simulink model "Lab7_Kho_Nguyen_Soh_AbdulKadir_simulink"  (R2021a)
settings: Solver=VariableStepAuto  StartTime=0.0  StopTime=10  MinStep=0.01  RelTol=1e-3
libraries: pid_lib x10, cstblocks x5
settings Model: Creator=fayeed  LastModifiedBy=kkqi_
settings SolverCC: AlgebraicLoopSolver=TrustRegion
settings DebuggingCC: SFMachineParentedDataDiag=warning

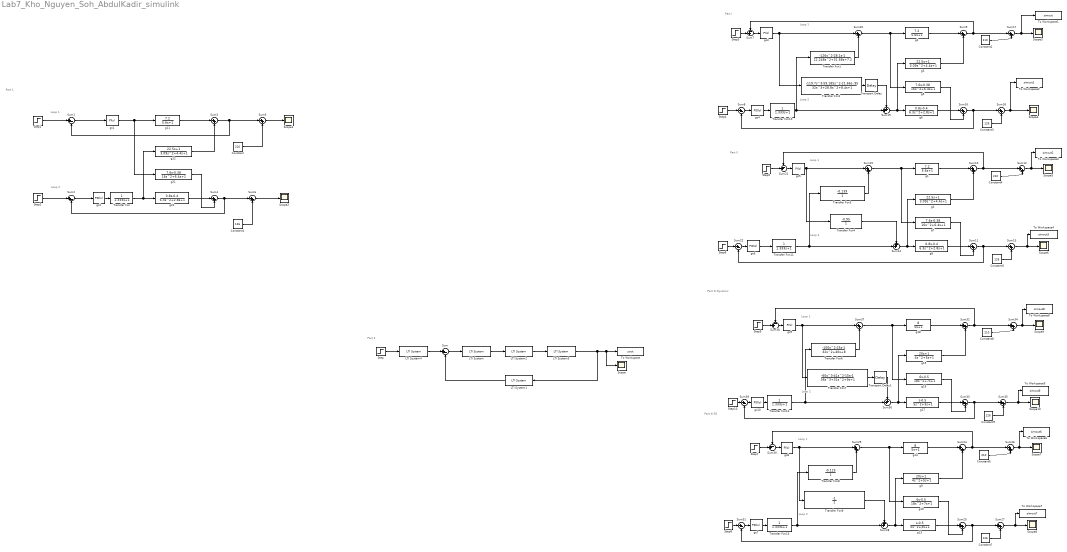
== system Lab7_Kho_Nguyen_Soh_AbdulKadir_simulink ==
  note: Part 1
  note: Part 3
  note: Loop 1
  note: Loop 2
  note: Part II
  note: Loop 2
  note: Loop 2
  note: Loop 1
  note: Loop 2
  note: Part I
  note: Loop 2
  note: Loop 1
  note: Loop 1
  note: Part III SS
  note: Part III Dynamic
  note: Loop 1
  Constant{,2,4,6,8} (5 alike) : Constant  Value=210
  Constant{1,3,5,7,9} (5 alike) : Constant  Value=126
  LTI System : cstblocks/LTI System  sys=Gc  IC=[]
  LTI System1 : cstblocks/LTI System  sys=WT  IC=[]
  LTI System2 : cstblocks/LTI System  sys=V  IC=[]
  LTI System3 : cstblocks/LTI System  sys=G  IC=[]
  LTI System4 : cstblocks/LTI System  sys=WT  IC=[]
  Scope{,1..10} (11 alike) : Scope
  Step : Step  Time=0  Before=[0,0,0]  After=[0,0,-10]  SampleTime=0
  Step{1,3,5,7,9} (5 alike) : Step  Time=0  After=15  SampleTime=0
  Step{2,4,6,8,10} (5 alike) : Step  Time=0  After=0  SampleTime=0
  Sum{,1..2,8,22,31,39} (7 alike) : Sum  Inputs=|+-
  Sum{3..6,9..13,15..18,20,24..27,29,32..35,37} (24 alike) : Sum  Inputs=|++
  Sum{14,19,28,36} (4 alike) : Sum  Inputs=++|
  Sum{7,21,30,38} (4 alike) : Sum  Inputs=-+|
  To Workspace : ToWorkspace  VariableName=yout  SampleTime=-1
  To Workspace1 : ToWorkspace  VariableName=simout  SampleTime=-1
  To Workspace2 : ToWorkspace  VariableName=simout1  SampleTime=-1
  To Workspace3 : ToWorkspace  VariableName=simout2  SampleTime=-1
  To Workspace4 : ToWorkspace  VariableName=simout3  SampleTime=-1
  To Workspace6 : ToWorkspace  VariableName=simout6  SampleTime=-1
  To Workspace7 : ToWorkspace  VariableName=simout7  SampleTime=-1
  To Workspace8 : ToWorkspace  VariableName=simout8  SampleTime=-1
  To Workspace9 : ToWorkspace  VariableName=simout9  SampleTime=-1
  Transfer Fcn{,10..13} (5 alike) : TransferFcn  Denominator=[1.333 1]
  Transfer Fcn1 : TransferFcn  Numerator=[-126 -28.1 -1]  Denominator=[22.248 31.68 7.2]
  Transfer Fcn2 : TransferFcn  Numerator=[-119.7 -59.185 -21.66 -.95]  Denominator=[32 28.8 8.4 1]
  Transfer Fcn3 : TransferFcn  Numerator=[-0.139]  Denominator=[1]
  Transfer Fcn4 : TransferFcn  Numerator=[-0.95]  Denominator=[1]
  Transfer Fcn6 : TransferFcn  Numerator=[-100 -25 -1]  Denominator=[32 40 8]
  Transfer Fcn7 : TransferFcn  Numerator=[-60 -41 -15 -1]  Denominator=[36 31 9 1]
  Transfer Fcn8 : TransferFcn  Numerator=[-0.125]  Denominator=[1]
  Transfer Fcn9 : TransferFcn  Numerator=[-1]  Denominator=[1]
  Transport Delay : TransportDelay  DelayTime=36
  Transport Delay1 : TransportDelay  DelayTime=20
  g1 : TransferFcn  Numerator=[7.2]  Denominator=[5.6 1]
  g10 : TransferFcn  Numerator=[6 -0.5]  Denominator=[18 7 1]
  g11 : TransferFcn  Numerator=[7.2]  Denominator=[5.6 1]
  g12 : TransferFcn  Numerator=[22.5 1]  Denominator=[3.09 4.4 1]
  g13 : TransferFcn  Numerator=[1 -0.5]  Denominator=[5 3 1 ]
  g14 : TransferFcn  Numerator=[8]  Denominator=[5 1]
  g15 : TransferFcn  Numerator=[20 1]  Denominator=[4 5 1]
  g16 : TransferFcn  Numerator=[6 -0.5]  Denominator=[18 7 1]
  g17 : TransferFcn  Numerator=[1 -0.5]  Denominator=[5 3 1 ]
  g18 : TransferFcn  Numerator=[8]  Denominator=[5 1]
  g2 : TransferFcn  Numerator=[7.2]  Denominator=[5.6 1]
  g21 : TransferFcn  Numerator=[7.6 -0.38]  Denominator=[16 6.4 1]
  g22 : TransferFcn  Numerator=[0.8 -0.4]  Denominator=[6.3 2.8 1]
  g3 : TransferFcn  Numerator=[22.5 1]  Denominator=[3.09 4.4 1]
  g4 : TransferFcn  Numerator=[22.5 1]  Denominator=[3.09 4.4 1]
  g5 : TransferFcn  Numerator=[7.6 -0.38]  Denominator=[16 6.4 1]
  g6 : TransferFcn  Numerator=[0.8 -0.4]  Denominator=[6.3 2.8 1]
  g7 : TransferFcn  Numerator=[7.6 -0.38]  Denominator=[16 6.4 1]
  g8 : TransferFcn  Numerator=[0.8 -0.4]  Denominator=[6.3 2.8 1]
  g9 : TransferFcn  Numerator=[20 1]  Denominator=[4 5 1]
  gc1 : pid_lib/PID Controller  Controller=PI  Form=Ideal  TimeDomain=Continuous-time  UseExternalTs=off  SampleTime=-1  IntegratorMethod=Forward Euler  FilterMethod=Forward Euler  ControllerParametersSource=internal  P=0.778  I=0.1779  D=0  UseFilter=on  N=100  TunerSelectOption=Transfer Function Based (PID Tuner App)  InitialConditionSource=internal  InitialConditionForIntegrator=0  InitialConditionForFilter=0  DifferentiatorICPrevScaledInput=0  ExternalReset=none  TrackingMode=off  Kt=1  LimitOutput=off  SatLimitsSource=internal  UpperSaturationLimit=inf  LowerSaturationLimit=-inf  LinearizeAsGain=on  AntiWindupMode=none  Kb=1  POutMin=[]  POutMax=[]  IOutMin=[]  IOutMax=[]  DOutMin=[]  DOutMax=[]  NOutMin=[]  NOutMax=[]  SumOutMin=[]  SumOutMax=[]  SaturationOutMin=[]  SaturationOutMax=[]  PParamMin=[]  PParamMax=[]  IParamMin=[]  IParamMax=[]  DParamMin=[]  DParamMax=[]  NParamMin=[]  NParamMax=[]  KbParamMin=[]  KbParamMax=[]  KtParamMin=[]  KtParamMax=[]  KbOutMin=[]  KbOutMax=[]  KtOutMin=[]  KtOutMax=[]  IntegratorOutMin=[]  IntegratorOutMax=[]  FilterOutMin=[]  FilterOutMax=[]  SumI1OutMin=[]  SumI1OutMax=[]  SumI2OutMin=[]  SumI2OutMax=[]  SumI3OutMin=[]  SumI3OutMax=[]  SumI4OutMin=[]  SumI4OutMax=[]  SumDOutMin=[]  SumDOutMax=[]  DifferentiatorOutMin=[]  DifferentiatorOutMax=[]  FilterDiffOutCoefMin=[]  FilterDiffOutCoefMax=[]  ReciprocalOutMin=[]  ReciprocalOutMax=[]  SumDenOutMin=[]  SumDenOutMax=[]  SumNumOutMin=[]  SumNumOutMax=[]  DivideOutMin=[]  DivideOutMax=[]  UdiffTsProdOutMin=[]  UdiffTsProdOutMax=[]  NTsProdOutMin=[]  NTsProdOutMax=[]  UintegralTsProdOutMin=[]  UintegralTsProdOutMax=[]  UngainTsProdOutMin=[]  UngainTsProdOutMax=[]  IntegratorContinuousStateAttributes=''  IntegratorStateMustResolveToSignalObject=off  IntegratorRTWStateStorageClass=Auto  FilterContinuousStateAttributes=''  FilterStateMustResolveToSignalObject=off  FilterRTWStateStorageClass=Auto  ParallelPVariant=Passthrough  IdealPVariant=InternalParameters  IVariant=InternalParameters  DVariant=Disabled  IntegratorVariant=Continuous  SatVariant=Disabled  AWVariant=Passthrough  PCopyVariant=Disabled  TRVariant=Disabled  FdbkBlocksVariant=Forward  IdealPFdbkVariant=Disabled  SatFdbkVariant=Disabled  DerivativeFilterVariant=Disabled  NVariant=Disabled  NCopyVariant=Disabled_SignalSpec  FilterICVariant=Disabled  IntegratorICVariant=InternalICs  ExternalResetVariant=Disabled  TRSumVariant=Passthrough  SumFdbkVariant=Disabled  SumVariant=Sum_PI  TsampFilterVariant=InternalTs  TsampNgainVariant=Passthrough  TsampIntegralVariant=Passthrough  ExternalSaturationOutDataTypeStr=Inherit: Same as second input
  gc{2,4,6..7,10} (5 alike) : pid_lib/PID Controller  Controller=PID  Form=Ideal  TimeDomain=Continuous-time  UseExternalTs=off  SampleTime=-1  IntegratorMethod=Forward Euler  FilterMethod=Forward Euler  ControllerParametersSource=internal  P=-0.778  I=0.357  D=2.25  UseFilter=on  N=100  TunerSelectOption=Transfer Function Based (PID Tuner App)  InitialConditionSource=internal  InitialConditionForIntegrator=0  InitialConditionForFilter=0  DifferentiatorICPrevScaledInput=0  ExternalReset=none  TrackingMode=off  Kt=1  LimitOutput=off  SatLimitsSource=internal  UpperSaturationLimit=inf  LowerSaturationLimit=-inf  LinearizeAsGain=on  AntiWindupMode=none  Kb=1  POutMin=[]  POutMax=[]  IOutMin=[]  IOutMax=[]  DOutMin=[]  DOutMax=[]  NOutMin=[]  NOutMax=[]  SumOutMin=[]  SumOutMax=[]  SaturationOutMin=[]  SaturationOutMax=[]  PParamMin=[]  PParamMax=[]  IParamMin=[]  IParamMax=[]  DParamMin=[]  DParamMax=[]  NParamMin=[]  NParamMax=[]  KbParamMin=[]  KbParamMax=[]  KtParamMin=[]  KtParamMax=[]  KbOutMin=[]  KbOutMax=[]  KtOutMin=[]  KtOutMax=[]  IntegratorOutMin=[]  IntegratorOutMax=[]  FilterOutMin=[]  FilterOutMax=[]  SumI1OutMin=[]  SumI1OutMax=[]  SumI2OutMin=[]  SumI2OutMax=[]  SumI3OutMin=[]  SumI3OutMax=[]  SumI4OutMin=[]  SumI4OutMax=[]  SumDOutMin=[]  SumDOutMax=[]  DifferentiatorOutMin=[]  DifferentiatorOutMax=[]  FilterDiffOutCoefMin=[]  FilterDiffOutCoefMax=[]  ReciprocalOutMin=[]  ReciprocalOutMax=[]  SumDenOutMin=[]  SumDenOutMax=[]  SumNumOutMin=[]  SumNumOutMax=[]  DivideOutMin=[]  DivideOutMax=[]  UdiffTsProdOutMin=[]  UdiffTsProdOutMax=[]  NTsProdOutMin=[]  NTsProdOutMax=[]  UintegralTsProdOutMin=[]  UintegralTsProdOutMax=[]  UngainTsProdOutMin=[]  UngainTsProdOutMax=[]  IntegratorContinuousStateAttributes=''  IntegratorStateMustResolveToSignalObject=off  IntegratorRTWStateStorageClass=Auto  FilterContinuousStateAttributes=''  FilterStateMustResolveToSignalObject=off  FilterRTWStateStorageClass=Auto  ParallelPVariant=Passthrough  IdealPVariant=InternalParameters  IVariant=InternalParameters  DVariant=InternalParameters  IntegratorVariant=Continuous  SatVariant=Disabled  AWVariant=Passthrough  PCopyVariant=Disabled  TRVariant=Disabled  FdbkBlocksVariant=Forward  IdealPFdbkVariant=Disabled  SatFdbkVariant=Disabled  DerivativeFilterVariant=ContFilter  NVariant=InternalParameters  NCopyVariant=Disabled  FilterICVariant=InternalICsFilter  IntegratorICVariant=InternalICs  ExternalResetVariant=Disabled  TRSumVariant=Passthrough  SumFdbkVariant=Disabled  SumVariant=Sum_PID  TsampFilterVariant=InternalTs  TsampNgainVariant=Passthrough  TsampIntegralVariant=Passthrough  ExternalSaturationOutDataTypeStr=Inherit: Same as second input
  gc3 : pid_lib/PID Controller  Controller=PI  Form=Ideal  TimeDomain=Continuous-time  UseExternalTs=off  SampleTime=-1  IntegratorMethod=Forward Euler  FilterMethod=Forward Euler  ControllerParametersSource=internal  P=0.778  I=0.1779  D=0  UseFilter=on  N=100  TunerSelectOption=Transfer Function Based (PID Tuner App)  InitialConditionSource=internal  InitialConditionForIntegrator=0  InitialConditionForFilter=0  DifferentiatorICPrevScaledInput=0  ExternalReset=none  TrackingMode=off  Kt=1  LimitOutput=off  SatLimitsSource=internal  UpperSaturationLimit=inf  LowerSaturationLimit=-inf  LinearizeAsGain=on  AntiWindupMode=none  Kb=1  POutMin=[]  POutMax=[]  IOutMin=[]  IOutMax=[]  DOutMin=[]  DOutMax=[]  NOutMin=[]  NOutMax=[]  SumOutMin=[]  SumOutMax=[]  SaturationOutMin=[]  SaturationOutMax=[]  PParamMin=[]  PParamMax=[]  IParamMin=[]  IParamMax=[]  DParamMin=[]  DParamMax=[]  NParamMin=[]  NParamMax=[]  KbParamMin=[]  KbParamMax=[]  KtParamMin=[]  KtParamMax=[]  KbOutMin=[]  KbOutMax=[]  KtOutMin=[]  KtOutMax=[]  IntegratorOutMin=[]  IntegratorOutMax=[]  FilterOutMin=[]  FilterOutMax=[]  SumI1OutMin=[]  SumI1OutMax=[]  SumI2OutMin=[]  SumI2OutMax=[]  SumI3OutMin=[]  SumI3OutMax=[]  SumI4OutMin=[]  SumI4OutMax=[]  SumDOutMin=[]  SumDOutMax=[]  DifferentiatorOutMin=[]  DifferentiatorOutMax=[]  FilterDiffOutCoefMin=[]  FilterDiffOutCoefMax=[]  ReciprocalOutMin=[]  ReciprocalOutMax=[]  SumDenOutMin=[]  SumDenOutMax=[]  SumNumOutMin=[]  SumNumOutMax=[]  DivideOutMin=[]  DivideOutMax=[]  UdiffTsProdOutMin=[]  UdiffTsProdOutMax=[]  NTsProdOutMin=[]  NTsProdOutMax=[]  UintegralTsProdOutMin=[]  UintegralTsProdOutMax=[]  UngainTsProdOutMin=[]  UngainTsProdOutMax=[]  IntegratorContinuousStateAttributes=''  IntegratorStateMustResolveToSignalObject=off  IntegratorRTWStateStorageClass=Auto  FilterContinuousStateAttributes=''  FilterStateMustResolveToSignalObject=off  FilterRTWStateStorageClass=Auto  ParallelPVariant=Passthrough  IdealPVariant=InternalParameters  IVariant=InternalParameters  DVariant=Disabled  IntegratorVariant=Continuous  SatVariant=Disabled  AWVariant=Passthrough  PCopyVariant=Disabled  TRVariant=Disabled  FdbkBlocksVariant=Forward  IdealPFdbkVariant=Disabled  SatFdbkVariant=Disabled  DerivativeFilterVariant=Disabled  NVariant=Disabled  NCopyVariant=Disabled_SignalSpec  FilterICVariant=Disabled  IntegratorICVariant=InternalICs  ExternalResetVariant=Disabled  TRSumVariant=Passthrough  SumFdbkVariant=Disabled  SumVariant=Sum_PI  TsampFilterVariant=InternalTs  TsampNgainVariant=Passthrough  TsampIntegralVariant=Passthrough  ExternalSaturationOutDataTypeStr=Inherit: Same as second input
  gc5 : pid_lib/PID Controller  Controller=PI  Form=Ideal  TimeDomain=Continuous-time  UseExternalTs=off  SampleTime=-1  IntegratorMethod=Forward Euler  FilterMethod=Forward Euler  ControllerParametersSource=internal  P=.0778  I=.1779  D=0  UseFilter=on  N=100  TunerSelectOption=Transfer Function Based (PID Tuner App)  InitialConditionSource=internal  InitialConditionForIntegrator=0  InitialConditionForFilter=0  DifferentiatorICPrevScaledInput=0  ExternalReset=none  TrackingMode=off  Kt=1  LimitOutput=off  SatLimitsSource=internal  UpperSaturationLimit=inf  LowerSaturationLimit=-inf  LinearizeAsGain=on  AntiWindupMode=none  Kb=1  POutMin=[]  POutMax=[]  IOutMin=[]  IOutMax=[]  DOutMin=[]  DOutMax=[]  NOutMin=[]  NOutMax=[]  SumOutMin=[]  SumOutMax=[]  SaturationOutMin=[]  SaturationOutMax=[]  PParamMin=[]  PParamMax=[]  IParamMin=[]  IParamMax=[]  DParamMin=[]  DParamMax=[]  NParamMin=[]  NParamMax=[]  KbParamMin=[]  KbParamMax=[]  KtParamMin=[]  KtParamMax=[]  KbOutMin=[]  KbOutMax=[]  KtOutMin=[]  KtOutMax=[]  IntegratorOutMin=[]  IntegratorOutMax=[]  FilterOutMin=[]  FilterOutMax=[]  SumI1OutMin=[]  SumI1OutMax=[]  SumI2OutMin=[]  SumI2OutMax=[]  SumI3OutMin=[]  SumI3OutMax=[]  SumI4OutMin=[]  SumI4OutMax=[]  SumDOutMin=[]  SumDOutMax=[]  DifferentiatorOutMin=[]  DifferentiatorOutMax=[]  FilterDiffOutCoefMin=[]  FilterDiffOutCoefMax=[]  ReciprocalOutMin=[]  ReciprocalOutMax=[]  SumDenOutMin=[]  SumDenOutMax=[]  SumNumOutMin=[]  SumNumOutMax=[]  DivideOutMin=[]  DivideOutMax=[]  UdiffTsProdOutMin=[]  UdiffTsProdOutMax=[]  NTsProdOutMin=[]  NTsProdOutMax=[]  UintegralTsProdOutMin=[]  UintegralTsProdOutMax=[]  UngainTsProdOutMin=[]  UngainTsProdOutMax=[]  IntegratorContinuousStateAttributes=''  IntegratorStateMustResolveToSignalObject=off  IntegratorRTWStateStorageClass=Auto  FilterContinuousStateAttributes=''  FilterStateMustResolveToSignalObject=off  FilterRTWStateStorageClass=Auto  ParallelPVariant=Passthrough  IdealPVariant=InternalParameters  IVariant=InternalParameters  DVariant=Disabled  IntegratorVariant=Continuous  SatVariant=Disabled  AWVariant=Passthrough  PCopyVariant=Disabled  TRVariant=Disabled  FdbkBlocksVariant=Forward  IdealPFdbkVariant=Disabled  SatFdbkVariant=Disabled  DerivativeFilterVariant=Disabled  NVariant=Disabled  NCopyVariant=Disabled_SignalSpec  FilterICVariant=Disabled  IntegratorICVariant=InternalICs  ExternalResetVariant=Disabled  TRSumVariant=Passthrough  SumFdbkVariant=Disabled  SumVariant=Sum_PI  TsampFilterVariant=InternalTs  TsampNgainVariant=Passthrough  TsampIntegralVariant=Passthrough  ExternalSaturationOutDataTypeStr=Inherit: Same as second input
  gc8 : pid_lib/PID Controller  Controller=PI  Form=Ideal  TimeDomain=Continuous-time  UseExternalTs=off  SampleTime=-1  IntegratorMethod=Forward Euler  FilterMethod=Forward Euler  ControllerParametersSource=internal  P=0.0778  I=0.178  D=0  UseFilter=on  N=100  TunerSelectOption=Transfer Function Based (PID Tuner App)  InitialConditionSource=internal  InitialConditionForIntegrator=0  InitialConditionForFilter=0  DifferentiatorICPrevScaledInput=0  ExternalReset=none  TrackingMode=off  Kt=1  LimitOutput=off  SatLimitsSource=internal  UpperSaturationLimit=inf  LowerSaturationLimit=-inf  LinearizeAsGain=on  AntiWindupMode=none  Kb=1  POutMin=[]  POutMax=[]  IOutMin=[]  IOutMax=[]  DOutMin=[]  DOutMax=[]  NOutMin=[]  NOutMax=[]  SumOutMin=[]  SumOutMax=[]  SaturationOutMin=[]  SaturationOutMax=[]  PParamMin=[]  PParamMax=[]  IParamMin=[]  IParamMax=[]  DParamMin=[]  DParamMax=[]  NParamMin=[]  NParamMax=[]  KbParamMin=[]  KbParamMax=[]  KtParamMin=[]  KtParamMax=[]  KbOutMin=[]  KbOutMax=[]  KtOutMin=[]  KtOutMax=[]  IntegratorOutMin=[]  IntegratorOutMax=[]  FilterOutMin=[]  FilterOutMax=[]  SumI1OutMin=[]  SumI1OutMax=[]  SumI2OutMin=[]  SumI2OutMax=[]  SumI3OutMin=[]  SumI3OutMax=[]  SumI4OutMin=[]  SumI4OutMax=[]  SumDOutMin=[]  SumDOutMax=[]  DifferentiatorOutMin=[]  DifferentiatorOutMax=[]  FilterDiffOutCoefMin=[]  FilterDiffOutCoefMax=[]  ReciprocalOutMin=[]  ReciprocalOutMax=[]  SumDenOutMin=[]  SumDenOutMax=[]  SumNumOutMin=[]  SumNumOutMax=[]  DivideOutMin=[]  DivideOutMax=[]  UdiffTsProdOutMin=[]  UdiffTsProdOutMax=[]  NTsProdOutMin=[]  NTsProdOutMax=[]  UintegralTsProdOutMin=[]  UintegralTsProdOutMax=[]  UngainTsProdOutMin=[]  UngainTsProdOutMax=[]  IntegratorContinuousStateAttributes=''  IntegratorStateMustResolveToSignalObject=off  IntegratorRTWStateStorageClass=Auto  FilterContinuousStateAttributes=''  FilterStateMustResolveToSignalObject=off  FilterRTWStateStorageClass=Auto  ParallelPVariant=Passthrough  IdealPVariant=InternalParameters  IVariant=InternalParameters  DVariant=Disabled  IntegratorVariant=Continuous  SatVariant=Disabled  AWVariant=Passthrough  PCopyVariant=Disabled  TRVariant=Disabled  FdbkBlocksVariant=Forward  IdealPFdbkVariant=Disabled  SatFdbkVariant=Disabled  DerivativeFilterVariant=Disabled  NVariant=Disabled  NCopyVariant=Disabled_SignalSpec  FilterICVariant=Disabled  IntegratorICVariant=InternalICs  ExternalResetVariant=Disabled  TRSumVariant=Passthrough  SumFdbkVariant=Disabled  SumVariant=Sum_PI  TsampFilterVariant=InternalTs  TsampNgainVariant=Passthrough  TsampIntegralVariant=Passthrough  ExternalSaturationOutDataTypeStr=Inherit: Same as second input
  gc9 : pid_lib/PID Controller  Controller=PI  Form=Ideal  TimeDomain=Continuous-time  UseExternalTs=off  SampleTime=-1  IntegratorMethod=Forward Euler  FilterMethod=Forward Euler  ControllerParametersSource=internal  P=.778  I=.1779  D=0  UseFilter=on  N=100  TunerSelectOption=Transfer Function Based (PID Tuner App)  InitialConditionSource=internal  InitialConditionForIntegrator=0  InitialConditionForFilter=0  DifferentiatorICPrevScaledInput=0  ExternalReset=none  TrackingMode=off  Kt=1  LimitOutput=off  SatLimitsSource=internal  UpperSaturationLimit=inf  LowerSaturationLimit=-inf  LinearizeAsGain=on  AntiWindupMode=none  Kb=1  POutMin=[]  POutMax=[]  IOutMin=[]  IOutMax=[]  DOutMin=[]  DOutMax=[]  NOutMin=[]  NOutMax=[]  SumOutMin=[]  SumOutMax=[]  SaturationOutMin=[]  SaturationOutMax=[]  PParamMin=[]  PParamMax=[]  IParamMin=[]  IParamMax=[]  DParamMin=[]  DParamMax=[]  NParamMin=[]  NParamMax=[]  KbParamMin=[]  KbParamMax=[]  KtParamMin=[]  KtParamMax=[]  KbOutMin=[]  KbOutMax=[]  KtOutMin=[]  KtOutMax=[]  IntegratorOutMin=[]  IntegratorOutMax=[]  FilterOutMin=[]  FilterOutMax=[]  SumI1OutMin=[]  SumI1OutMax=[]  SumI2OutMin=[]  SumI2OutMax=[]  SumI3OutMin=[]  SumI3OutMax=[]  SumI4OutMin=[]  SumI4OutMax=[]  SumDOutMin=[]  SumDOutMax=[]  DifferentiatorOutMin=[]  DifferentiatorOutMax=[]  FilterDiffOutCoefMin=[]  FilterDiffOutCoefMax=[]  ReciprocalOutMin=[]  ReciprocalOutMax=[]  SumDenOutMin=[]  SumDenOutMax=[]  SumNumOutMin=[]  SumNumOutMax=[]  DivideOutMin=[]  DivideOutMax=[]  UdiffTsProdOutMin=[]  UdiffTsProdOutMax=[]  NTsProdOutMin=[]  NTsProdOutMax=[]  UintegralTsProdOutMin=[]  UintegralTsProdOutMax=[]  UngainTsProdOutMin=[]  UngainTsProdOutMax=[]  IntegratorContinuousStateAttributes=''  IntegratorStateMustResolveToSignalObject=off  IntegratorRTWStateStorageClass=Auto  FilterContinuousStateAttributes=''  FilterStateMustResolveToSignalObject=off  FilterRTWStateStorageClass=Auto  ParallelPVariant=Passthrough  IdealPVariant=InternalParameters  IVariant=InternalParameters  DVariant=Disabled  IntegratorVariant=Continuous  SatVariant=Disabled  AWVariant=Passthrough  PCopyVariant=Disabled  TRVariant=Disabled  FdbkBlocksVariant=Forward  IdealPFdbkVariant=Disabled  SatFdbkVariant=Disabled  DerivativeFilterVariant=Disabled  NVariant=Disabled  NCopyVariant=Disabled_SignalSpec  FilterICVariant=Disabled  IntegratorICVariant=InternalICs  ExternalResetVariant=Disabled  TRSumVariant=Passthrough  SumFdbkVariant=Disabled  SumVariant=Sum_PI  TsampFilterVariant=InternalTs  TsampNgainVariant=Passthrough  TsampIntegralVariant=Passthrough  ExternalSaturationOutDataTypeStr=Inherit: Same as second input
  wires:
  LTI System4/1 -> Sum/1
  Step/1 -> LTI System4/1
  Sum/1 -> LTI System/1
  LTI System/1 -> LTI System2/1
  LTI System2/1 -> LTI System3/1
  LTI System3/1 -> LTI System1/1, Scope/1, To Workspace/1
  LTI System1/1 -> Sum/2
  g12/1 -> Sum3/2
  Sum5/1 -> Scope1/1
  Step2/1 -> Sum2/1
  Sum2/1 -> gc2/1
  Step1/1 -> Sum1/1
  Sum3/1 -> Sum5/1, Sum1/2
  g21/1 -> Sum4/2
  gc2/1 -> Transfer Fcn/1
  Constant/1 -> Sum5/2
  g22/1 -> Sum4/1
  Sum4/1 -> Sum6/1, Sum2/2
  Constant1/1 -> Sum6/2
  Sum6/1 -> Scope2/1
  gc1/1 -> g21/1, g11/1
  g11/1 -> Sum3/1
  Transfer Fcn/1 -> g12/1, g22/1
  Sum1/1 -> gc1/1
  g17/1 -> Sum33/1
  Sum29/1 -> g10/1, g14/1
  Transfer Fcn9/1 -> Sum28/1
  Sum24/1 -> Sum26/1, Sum30/1
  g9/1 -> Sum24/2
  Constant7/1 -> Sum27/2
  Constant6/1 -> Sum26/2
  Step7/1 -> Sum30/2
  Step10/1 -> Sum39/1
  Step3/1 -> Sum7/2
  Sum28/1 -> g9/1, g13/1
  Sum13/1 -> To Workspace4/1, Scope6/1
  Transfer Fcn11/1 -> Sum14/2, Transfer Fcn3/1
  g18/1 -> Sum32/1
  g13/1 -> Sum25/1
  Constant8/1 -> Sum34/2
  g3/1 -> Sum9/2
  Sum10/1 -> Sum12/1, Sum21/1
  Constant4/1 -> Sum12/2
  Sum17/1 -> To Workspace1/1, Scope3/1
  Sum9/1 -> Sum17/1, Sum7/1
  Step5/1 -> Sum21/2
  Sum16/1 -> Sum18/1, Sum8/2
  Sum15/1 -> g7/1, g1/1
  Sum25/1 -> Sum27/1, Sum31/2
  Sum14/1 -> g4/1, g8/1
  Transfer Fcn2/1 -> Transport Delay/1
  g2/1 -> Sum9/1
  Transport Delay/1 -> Sum19/1
  Constant2/1 -> Sum17/2
  g5/1 -> Sum16/2
  Constant3/1 -> Sum18/2
  Sum8/1 -> gc4/1
  Sum7/1 -> gc3/1
  g4/1 -> Sum10/2
  Constant9/1 -> Sum35/2
  g8/1 -> Sum11/1
  Sum37/1 -> g16/1, g18/1
  Transfer Fcn8/1 -> Sum29/2
  Sum34/1 -> To Workspace8/1, Scope9/1
  Step4/1 -> Sum8/1
  Transfer Fcn1/1 -> Sum20/2
  g7/1 -> Sum11/2
  Sum22/1 -> gc6/1
  Sum39/1 -> gc10/1
  Sum12/1 -> To Workspace3/1, Scope5/1
  Step8/1 -> Sum31/1
  g1/1 -> Sum10/1
  Sum21/1 -> gc5/1
  Sum11/1 -> Sum13/1, Sum22/2
  gc8/1 -> Transfer Fcn9/1, Sum29/1
  gc5/1 -> Sum15/1, Transfer Fcn4/1
  g15/1 -> Sum32/2
  Sum27/1 -> To Workspace7/1, Scope8/1
  Sum31/1 -> gc7/1
  Constant5/1 -> Sum13/2
  g10/1 -> Sum25/2
  Sum38/1 -> gc9/1
  Step9/1 -> Sum38/2
  Sum33/1 -> Sum35/1, Sum39/2
  g16/1 -> Sum33/2
  Sum36/1 -> g15/1, g17/1
  Sum19/1 -> g3/1, g6/1
  Transfer Fcn3/1 -> Sum15/2
  Sum18/1 -> Scope4/1, To Workspace2/1
  Sum20/1 -> g5/1, g2/1
  g6/1 -> Sum16/1
  Sum32/1 -> Sum34/1, Sum38/1
  Step6/1 -> Sum22/1
  Transfer Fcn6/1 -> Sum37/2
  gc9/1 -> Transfer Fcn7/1, Sum37/1
  Transfer Fcn10/1 -> Sum19/2, Transfer Fcn1/1
  g14/1 -> Sum24/1
  gc4/1 -> Transfer Fcn10/1
  Transport Delay1/1 -> Sum36/1
  gc7/1 -> Transfer Fcn13/1
  Transfer Fcn12/1 -> Sum36/2, Transfer Fcn6/1
  Sum30/1 -> gc8/1
  Sum26/1 -> To Workspace6/1, Scope7/1
  Sum35/1 -> To Workspace9/1, Scope10/1
  gc10/1 -> Transfer Fcn12/1
  Transfer Fcn13/1 -> Transfer Fcn8/1, Sum28/2
  Transfer Fcn4/1 -> Sum14/1
  gc6/1 -> Transfer Fcn11/1
  gc3/1 -> Transfer Fcn2/1, Sum20/1
  Transfer Fcn7/1 -> Transport Delay1/1
